simulink model "servoDrive"  (R2019b)
settings: Solver=FixedStepAuto  StartTime=0.0  StopTime=inf  FixedStep=0.5  RelTol=1e-3  EnableMultiTasking=on
libraries: arduinolib x4
settings Model: SimulationMode=external  SILPILModeSetting=veronly  ExtModeTrigDuration=2  Creator=covasanvictor  LastModifiedBy=covasanvictor
settings OptimizationCC: EnhancedBackFolding=on  PassReuseOutputArgsAs=Individual arguments  ZeroExternalMemoryAtStartup=off  ZeroInternalMemoryAtStartup=off  MaxStackSize=64  OptimizeBlockOrder=speed  DifferentSizesBufferReuse=on  OptimizationCustomize=off  EfficientTunableParamExpr=on
settings DebuggingCC: ParameterTunabilityLossMsg=error
settings HardwareCC: ProdBitPerInt=16  ProdBitPerPointer=16  ProdBitPerSizeT=16  ProdBitPerPtrDiffT=16  ProdLargestAtomicFloat=None  ProdWordSize=8  ProdHWDeviceType=Atmel->AVR  UseEmbeddedCoderFeatures=off  UseSimulinkCoderFeatures=off
settings SFSimCC: MATLABDynamicMemAlloc=off
settings RTWCC: SystemTargetFile=ert.tlc  HardwareBoard=Arduino Uno  TLCOptions=-aInlineSetEventsForThisBaseRateFcn=TLC_FALSE -aSuppressMultiTaskScheduler=TLC_FALSE -aRateBasedStepFcn=1  TemplateMakefile=ert_default_tmf  GenerateReport=on  Toolchain=Arduino AVR  BuildConfiguration=Faster Runs  IncludeHyperlinkInReport=on  LaunchReport=on  GenerateTraceInfo=on  GenerateTraceReport=on  GenerateTraceReportSl=on  GenerateTraceReportSf=on  GenerateTraceReportEml=on
settings CodeAppCC: ForceParamTrailComments=on  IgnoreCustomStorageClasses=off  OperatorAnnotations=on  SimulinkDataObjDesc=on  SFDataObjDesc=on  InsertBlockDesc=on
settings ERTTargetCC: SupportContinuousTime=on  SupportNonInlinedSFcns=on  SupportVariableSizeSignals=on  ExtModeStaticAllocSize=250

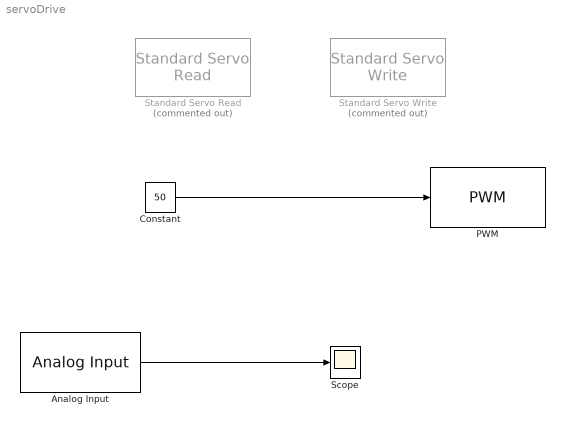
== system servoDrive ==
  Analog Input : arduinolib/Analog Input  pinNumber=0  ReadResultsOnly=off  ConversionTriggerSource=Software  ExternalTriggerType=uint32(0)  OutputDataType=uint16  EnableConversionCompleteNotify=off  EnableOuputStatus=off  SampleTime=-1  blockPlatform=arduino
  Constant : Constant  Value=50
  PWM : arduinolib/PWM  pinNumber=3  EnableInputFrequency=off  InitialFrequency=2000  InitialDutyCycle=0  NotificationType=None  blockPlatform=arduino
  Scope : Scope
  Standard Servo Read : arduinolib/Standard Servo Read  Commented=on  pinNumber=2  SampleTime=0.1  ServoIndex=0  blockPlatform=ARDUINO
      settings: SourceProductName=Simulink Support Package for Arduino Hardware  SourceProductBaseCode=ARDUINO
  Standard Servo Write : arduinolib/Standard Servo Write  Commented=on  pinNumber=3  ServoIndex=0  blockPlatform=ARDUINO
      settings: SourceProductName=Simulink Support Package for Arduino Hardware
  wires:
  Analog Input/1 -> Scope/1
  Constant/1 -> PWM/1
